simulink model "LQservo_ClosedLoopBallandBeam"  (R2019a)
settings: Solver=VariableStepAuto  StartTime=0.0  StopTime=45.0  RelTol=1e-3
values from neighbouring files (symbols this model uses):
  A = [0   1   0   0 ... (first row only)    [BallandBeamModeling.m]
  B = [0;  b1; 0;  0]    [BallandBeamModeling.m]
  initTheta = 30/180*pi    (= 0.523598775598)    [BallandBeamModeling.m]
  wantx1 = 5    [BallandBeamModeling.m]
  wantx2 = 10    [BallandBeamModeling.m]
undefined symbols (not defined in the file or in its folder): K_servo
settings Model: Creator=xde12  LastModifiedBy=xde12

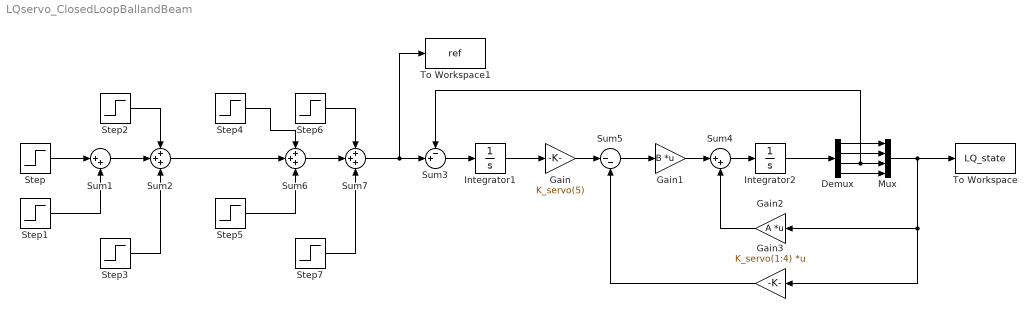
== system LQservo_ClosedLoopBallandBeam ==
  Demux : Demux
  Gain : Gain  Gain=K_servo(5)
  Gain1 : Gain  Gain=B  Multiplication=Matrix(K*u)
  Gain2 : Gain  Gain=A  Multiplication=Matrix(K*u)
  Gain3 : Gain  Gain=K_servo(1:4)  Multiplication=Matrix(K*u)
  Integrator1 : Integrator  InitialCondition=initTheta
  Integrator2 : Integrator
  Mux : Mux
  Step : Step  Time=5  After=wantx1  SampleTime=0
  Step1 : Step  Time=10  After=-wantx1  SampleTime=0
  Step2 : Step  Time=15  After=-wantx1  SampleTime=0
  Step3 : Step  Time=20  After=wantx1  SampleTime=0
  Step4 : Step  Time=25  After=wantx2  SampleTime=0
  Step5 : Step  Time=30  After=-wantx2  SampleTime=0
  Step6 : Step  Time=35  After=-wantx2  SampleTime=0
  Step7 : Step  Time=40  After=wantx2  SampleTime=0
  Sum1 : Sum  Inputs=|++
  Sum2 : Sum  Inputs=+++
  Sum3 : Sum  Inputs=-+|
  Sum4 : Sum  Inputs=|++
  Sum5 : Sum  Inputs=|--
  Sum6 : Sum  Inputs=+++
  Sum7 : Sum  Inputs=+++
  To Workspace : ToWorkspace  VariableName=LQ_state  SampleTime=-1
  To Workspace1 : ToWorkspace  VariableName=ref  SampleTime=-1
  wires:
  Sum3/1 -> Integrator1/1
  Integrator1/1 -> Gain/1
  Gain1/1 -> Sum4/1
  Sum4/1 -> Integrator2/1
  Gain/1 -> Sum5/1
  Gain2/1 -> Sum4/2
  Integrator2/1 -> Demux/1
  Demux/1 -> Mux/1
  Demux/2 -> Mux/2
  Demux/3 -> Sum3/1, Mux/3
  Demux/4 -> Mux/4
  Mux/1 -> To Workspace/1, Gain3/1, Gain2/1
  Gain3/1 -> Sum5/2
  Sum5/1 -> Gain1/1
  Step3/1 -> Sum2/3
  Sum2/1 -> Sum6/2
  Sum1/1 -> Sum2/2
  Step2/1 -> Sum2/1
  Step7/1 -> Sum7/3
  Step1/1 -> Sum1/2
  Step4/1 -> Sum6/1
  Step/1 -> Sum1/1
  Step6/1 -> Sum7/1
  Step5/1 -> Sum6/3
  Sum6/1 -> Sum7/2
  Sum7/1 -> To Workspace1/1, Sum3/2
